simulink model "BoundedTorqueControl2012b"  (Simulink 8.0)
settings: Solver=FixedStepDiscrete  StartTime=0.0  StopTime=CONFIG.SIMULATION_TIME  FixedStep=CONFIG.Ts  RelTol=1e-3
InitFcn:
  | cd(fileparts(which(bdroot)));
  | init_BoundedTorqueControl;
undefined symbols (not defined in the file or in its folder): CONFIG, DiscIntNeverNeededParam, model, ROBOT_DOF
libraries: WBToolboxLibrary x10
settings Model: Creator=marie  LastModifiedBy=DanielePucci  CovModelRefEnable=off
settings DataIOCC: SaveFormat=StructureWithTime
settings OptimizationCC: ExpressionDepthLimit=128
settings DebuggingCC: UnderspecifiedInitializationDetection=Simplified  MergeDetectMultiDrivingBlocksExec=error  SolverPrmCheckMsg=none  FrameProcessingCompatibilityMsg=error  StateNameClashWarn=none
settings HardwareCC: ProdBitPerPointer=64  ProdLargestAtomicFloat=Float  ProdIntDivRoundTo=Zero  ProdEndianess=LittleEndian  ProdHWDeviceType=Specified
settings CodeAppCC: CustomSymbolStrType=$N$R$M_T
settings GRTTargetCC: CodeReplacementLibrary=C89/C90 (ANSI)  GeneratePreprocessorConditionals=Use local settings

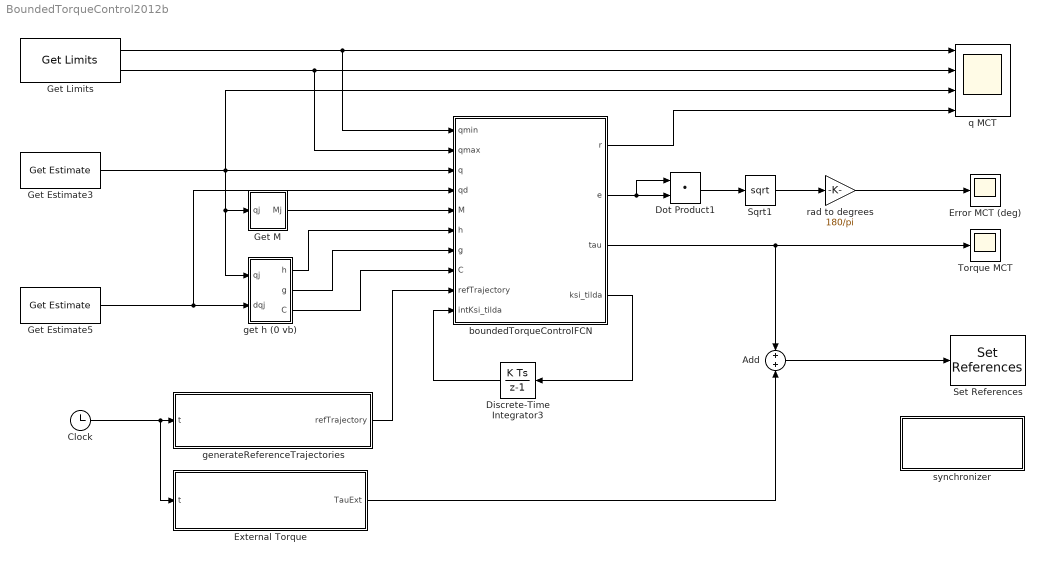
== system BoundedTorqueControl2012b ==
  Add : Sum
  Clock : Clock
  Discrete-Time Integrator3 : DiscreteIntegrator  InitialCondition=zeros(ROBOT_DOF,1)  InitialConditionMode=State only (most efficient)  SampleTime=CONFIG.Ts  ICPrevOutput=DiscIntNeverNeededParam  ICPrevScaledInput=DiscIntNeverNeededParam
  Dot Product1 : DotProduct  InputSameDT=on  OutDataTypeStr=Inherit: Inherit via internal rule
  Error MCT (deg) : Scope
      settings: TimeRange=auto  MaxDataPoints=5000  SaveToWorkspace=off  YMin=-2.39029  YMax=21.66052  SampleTime=-1
  External Torque : MATLAB Function  TreatAsAtomicUnit=on
      settings: PermitHierarchicalResolution=ParametersOnly
  Get Estimate3 : WBToolboxLibrary/wholeBodyStates/Get Estimate  estimateType=Joints Position  robotName=WBT_robotName  localName=WBT_modelName  wbiFile=WBT_wbiFilename  wbiList=WBT_wbiList
  Get Estimate5 : WBToolboxLibrary/wholeBodyStates/Get Estimate  estimateType=Joints Velocity  robotName=WBT_robotName  localName=WBT_modelName  wbiFile=WBT_wbiFilename  wbiList=WBT_wbiList
  Get Limits : WBToolboxLibrary/wholeBodyStates/Get Limits  limitsType=Position  robotName=WBT_robotName  localName=WBT_modelName  wbiFile=WBT_wbiFilename  wbiList=WBT_wbiList
  Get M : Subsystem
  Set References : WBToolboxLibrary/wholeBodyActuators/Set References  controlType=Torque  robotName=WBT_robotName  localName=WBT_modelName  wbiFile=WBT_wbiFilename  wbiList=WBT_wbiList
  Sqrt1 : Sqrt  SaturateOnIntegerOverflow=on
  Torque MCT : Scope
      settings: TimeRange=auto  MaxDataPoints=5000  SaveToWorkspace=off  SaveName=ScopeData2  YMin=-1131.02545  YMax=375.48726  SampleTime=-1
  boundedTorqueControlFCN : MATLAB Function  TreatAsAtomicUnit=on
      settings: PermitHierarchicalResolution=ParametersOnly
  generateReferenceTrajectories : MATLAB Function  TreatAsAtomicUnit=on
      settings: PermitHierarchicalResolution=ParametersOnly
  get h (0 vb) : Subsystem
  q MCT : Scope  NumInputPorts=4
      settings: TimeRange=auto  MaxDataPoints=5000  SaveToWorkspace=off  SaveName=ScopeData3  YMin=-2.50455~-5~-5~-5  YMax=0.72431~5~5~5  SampleTime=-1
  rad to degrees : Gain  Gain=180/pi
  synchronizer : Subsystem
      mask Display: disp('SYNCHRONIZER')
  wires:
  Get Estimate3/1 -> get h (0 vb)/1(qj), Get M/1(qj), q MCT/3, boundedTorqueControlFCN/3(q)
  Get Estimate5/1 -> boundedTorqueControlFCN/4(qd), get h (0 vb)/2(dqj)
  Get M/1(Mj) -> boundedTorqueControlFCN/5(M)
  get h (0 vb)/1(h) -> boundedTorqueControlFCN/6(h)
  Get Limits/2 -> boundedTorqueControlFCN/2(qmax), q MCT/2
  Get Limits/1 -> boundedTorqueControlFCN/1(qmin), q MCT/1
  boundedTorqueControlFCN/3(tau) -> Torque MCT/1, Add/1
  boundedTorqueControlFCN/4(ksi_tilda) -> Discrete-Time Integrator3/1
  Discrete-Time Integrator3/1 -> boundedTorqueControlFCN/10(intKsi_tilda)
  boundedTorqueControlFCN/2(e) -> Dot Product1/1, Dot Product1/2
  Dot Product1/1 -> Sqrt1/1
  Sqrt1/1 -> rad to degrees/1
  rad to degrees/1 -> Error MCT (deg)/1
  Add/1 -> Set References/1
  Clock/1 -> External Torque/1(t), generateReferenceTrajectories/1(t)
  External Torque/1(TauExt) -> Add/2
  generateReferenceTrajectories/1(refTrajectory) -> boundedTorqueControlFCN/9(refTrajectory)
  boundedTorqueControlFCN/1(r) -> q MCT/4
  get h (0 vb)/2(g) -> boundedTorqueControlFCN/7(g)
  get h (0 vb)/3(C) -> boundedTorqueControlFCN/8(C)

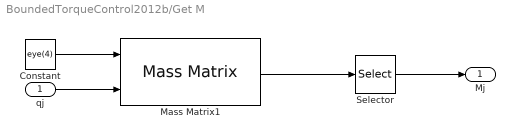
== system BoundedTorqueControl2012b/Get M ==
  qj : Inport
  Constant : Constant  Value=eye(4)
  Mass Matrix1 : WBToolboxLibrary/wholeBodyModel/Dynamics/Mass Matrix  robotName=WBT_robotName  localName=WBT_modelName  wbiFile=WBT_wbiFilename  wbiList=WBT_wbiList
  Selector : Selector  NumberOfDimensions=2  InputPortWidth=3  IndexOptions=Index vector (dialog),Index vector (dialog)  Indices=[7:6+ROBOT_DOF],[7:6+ROBOT_DOF]  OutputSizes=1,1
  Mj : Outport
  wires:
  Selector/1 -> Mj/1
  qj/1 -> Mass Matrix1/2
  Mass Matrix1/1 -> Selector/1
  Constant/1 -> Mass Matrix1/1

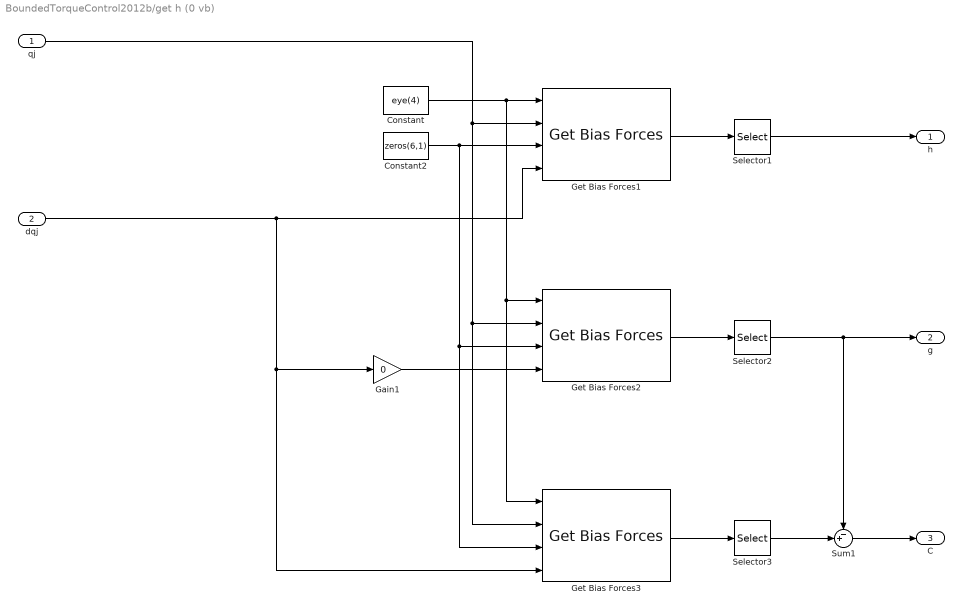
== system BoundedTorqueControl2012b/get h (0 vb) ==
  qj : Inport
  dqj : Inport  Port=2
  Constant : Constant  Value=eye(4)
  Constant2 : Constant  Value=zeros(6,1)
  Gain1 : Gain  Gain=0
  Get Bias Forces1 : WBToolboxLibrary/wholeBodyModel/Dynamics/Get Bias Forces  robotName=WBT_robotName  localName=WBT_modelName  wbiFile=WBT_wbiFilename  wbiList=WBT_wbiList  explicitGravity=off
  Get Bias Forces2 : WBToolboxLibrary/wholeBodyModel/Dynamics/Get Bias Forces  robotName=WBT_robotName  localName=WBT_modelName  wbiFile=WBT_wbiFilename  wbiList=WBT_wbiList  explicitGravity=off
  Get Bias Forces3 : WBToolboxLibrary/wholeBodyModel/Dynamics/Get Bias Forces  robotName=WBT_robotName  localName=WBT_modelName  wbiFile=WBT_wbiFilename  wbiList=WBT_wbiList  explicitGravity=off
  Selector1 : Selector  InputPortWidth=ROBOT_DOF+6  IndexOptions=Index vector (dialog)  Indices=[7:ROBOT_DOF+6]  OutputSizes=1
  Selector2 : Selector  InputPortWidth=ROBOT_DOF+6  IndexOptions=Index vector (dialog)  Indices=[7:ROBOT_DOF+6]  OutputSizes=1
  Selector3 : Selector  InputPortWidth=ROBOT_DOF+6  IndexOptions=Index vector (dialog)  Indices=[7:ROBOT_DOF+6]  OutputSizes=1
  Sum1 : Sum  Inputs=-+|
  h : Outport
  g : Outport  Port=2
  C : Outport  Port=3
  wires:
  Get Bias Forces1/1 -> Selector1/1
  qj/1 -> Get Bias Forces3/2, Get Bias Forces2/2, Get Bias Forces1/2
  Constant2/1 -> Get Bias Forces1/3, Get Bias Forces3/3, Get Bias Forces2/3
  Gain1/1 -> Get Bias Forces2/4
  Get Bias Forces2/1 -> Selector2/1
  Selector2/1 -> Sum1/1, g/1
  Get Bias Forces3/1 -> Selector3/1
  Selector3/1 -> Sum1/2
  Sum1/1 -> C/1
  dqj/1 -> Get Bias Forces1/4, Get Bias Forces3/4, Gain1/1
  Selector1/1 -> h/1
  Constant/1 -> Get Bias Forces2/1, Get Bias Forces3/1, Get Bias Forces1/1

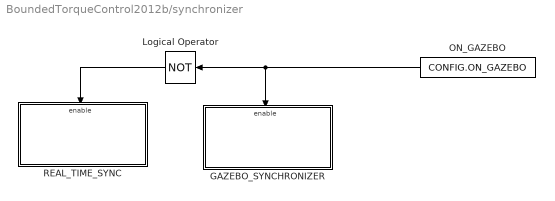
== system BoundedTorqueControl2012b/synchronizer ==
  GAZEBO_SYNCHRONIZER : Subsystem
  Logical Operator : Logic  Operator=NOT  AllPortsSameDT=off  OutDataTypeStr=boolean
  "ON_GAZEBO " : Constant  Value=CONFIG.ON_GAZEBO
  REAL_TIME_SYNC : Subsystem
  wires:
  Logical Operator/1 -> REAL_TIME_SYNC/Enable
  "ON_GAZEBO "/1 -> GAZEBO_SYNCHRONIZER/Enable, Logical Operator/1

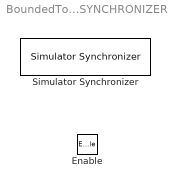
== system BoundedTorqueControl2012b/synchronizer/GAZEBO_SYNCHRONIZER ==
  Enable : EnablePort
  Simulator Synchronizer : WBToolboxLibrary/Utilities/Simulator Synchronizer  period=CONFIG.Ts  serverPortName='/clock/rpc'  clientPortName='/WBT_synchronizer/rpc:o'

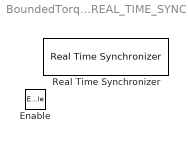
== system BoundedTorqueControl2012b/synchronizer/REAL_TIME_SYNC ==
  Enable : EnablePort
  Real Time Synchronizer : WBToolboxLibrary/Utilities/Real Time Synchronizer  period=CONFIG.Ts

== matlab function boundedTorqueControlFCN ==
  data: r output double; ROBOT_DOF parameter double; model parameter double; qmin input double; qmax input double; q input double; qd input double; M input double; h input double; g input double; C input double; refTrajectory input double; intKsi_tilda input double; e output double; tau output double; ksi_tilda output double
function [r, e, tau, ksi_tilda] = boundedJointEvolutionControlFCN(ROBOT_DOF, model, qmin, qmax, q, qd, M, h, g, C, refTrajectory, intKsi_tilda)


[r, e, tau, ksi_tilda] = boundedJointEvolutionControl(ROBOT_DOF, model, qmin, qmax, q, qd, M, h, g, C, refTrajectory, intKsi_tilda);

== matlab function generateReferenceTrajectories ==
  data: refTrajectory output double; t input double; model parameter double
function refTrajectory  = generateReferenceTrajectoriesFCN(t, model)

refTrajectory  = generateReferenceTrajectories(t, model);

== matlab function External Torque ==
  data: TauExt output double; t input double; model parameter double
function TauExt = applyExternTorqueFCN(t, model)

TauExt = applyExternTorque(t, model);
